simulink library "Lib_Cntrl_SetPointCntrlPI_TMATS"  (R2015a)
settings: Solver=ode45  StartTime=0.0  StopTime=10.0  RelTol=1e-3
Description:
  | Thomas Modules
settings Model: Creator=jwchapm2  LastModifiedBy=jwchapm2
settings OptimizationCC: ExpressionDepthLimit=2147483647
settings DebuggingCC: UnderspecifiedInitializationDetection=Classic  MergeDetectMultiDrivingBlocksExec=none  SolverPrmCheckMsg=warning  StateNameClashWarn=warning

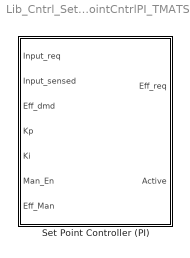
== system Lib_Cntrl_SetPointCntrlPI_TMATS ==
  Set Point Controller (PI) : Subsystem  mask(T-MATS: Set Point Controller (PI)){PI_IC_M=70, WGain_M=400, Ts_M=0.1}
      mask prompts: PI_IC_M "PI_IC_M - PI initial condition"; WGain_M "WGain_M - Windup protection gain"; Ts_M "Ts_M - Sample time"
      mask help: This block contains a PI controller with anti-windup protection. Gains, Kp and Ki, are define external to the block.
      mask Help: web(which('Control_TMATS_SPCPI.html'),'-helpbrowser')

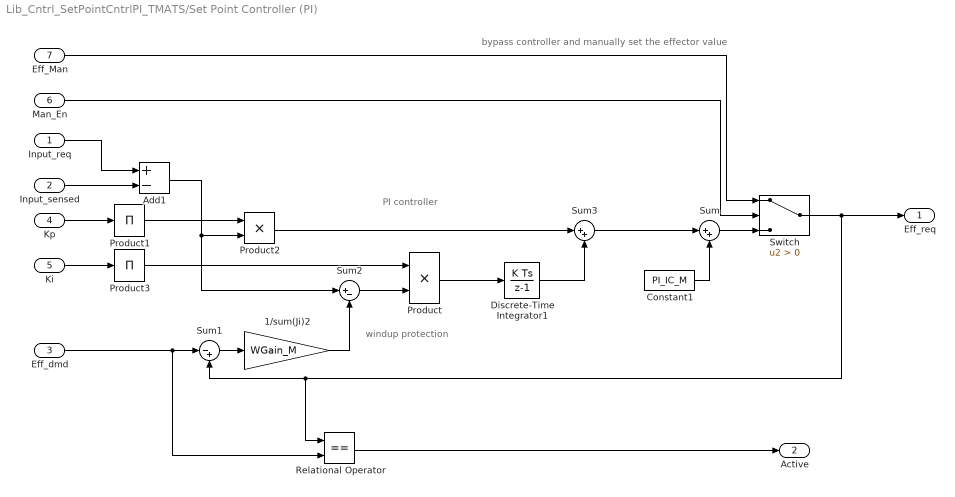
== system Lib_Cntrl_SetPointCntrlPI_TMATS/Set Point Controller (PI) ==
  note: bypass controller and manually set the effector value
  note: windup protection
  note: PI controller
  Input_req : Inport
  Input_sensed : Inport  Port=2
  Eff_dmd : Inport  Port=3
  Kp : Inport  Port=4
  Ki : Inport  Port=5
  Man_En : Inport  Port=6
  Eff_Man : Inport  Port=7
  1/sum(Ji)2 : Gain  Gain=WGain_M  SaturateOnIntegerOverflow=on  OutDataTypeStr=Inherit: Same as input  ParamDataTypeStr=Inherit: Same as input
  Add1 : Sum  Inputs=+-
  Constant1 : Constant  Value=PI_IC_M
  Discrete-Time Integrator1 : DiscreteIntegrator  InitialConditionSetting=State (most efficient)  SampleTime=Ts_M
  Product : Product
  Product1 : Product  Inputs=1
  Product2 : Product
  Product3 : Product  Inputs=1
  Relational Operator : RelationalOperator  Operator===  OutDataTypeStr=boolean
  Sum : Sum  Inputs=|++
  Sum1 : Sum  Inputs=|-+
  Sum2 : Sum  Inputs=|+-
  Sum3 : Sum  Inputs=|++
  Switch : Switch  Criteria=u2 > Threshold
  Eff_req : Outport
  Active : Outport  Port=2
  wires:
  Add1/1 -> Product2/2, Sum2/1
  Input_sensed/1 -> Add1/2
  Product2/1 -> Sum3/1
  Input_req/1 -> Add1/1
  Discrete-Time Integrator1/1 -> Sum3/2
  Switch/1 -> Relational Operator/1, Sum1/2, Eff_req/1
  Eff_dmd/1 -> Relational Operator/2, Sum1/1
  Sum1/1 -> 1/sum(Ji)2/1
  1/sum(Ji)2/1 -> Sum2/2
  Sum2/1 -> Product/2
  Product/1 -> Discrete-Time Integrator1/1
  Ki/1 -> Product3/1
  Relational Operator/1 -> Active/1
  Kp/1 -> Product1/1
  Product1/1 -> Product2/1
  Product3/1 -> Product/1
  Sum/1 -> Switch/3
  Sum3/1 -> Sum/1
  Constant1/1 -> Sum/2
  Eff_Man/1 -> Switch/1
  Man_En/1 -> Switch/2
